simulink model "ResidualAware_TruckSim_Cosim"  (R2022b)
settings: Solver=FixedStepDiscrete  StartTime=0.0  StopTime=130  FixedStep=0.04  RelTol=1e-3
undefined symbols (not defined in the file or in its folder): ra_ego0, ra_P
settings Model: Creator=fjb  LastModifiedBy=fjb

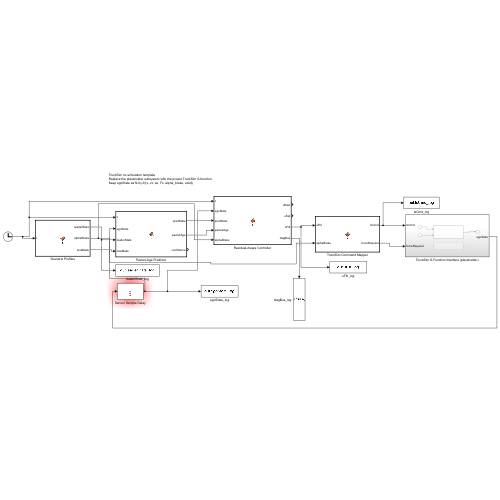
[thumbnail: Simulink's stored preview of the top-level diagram]
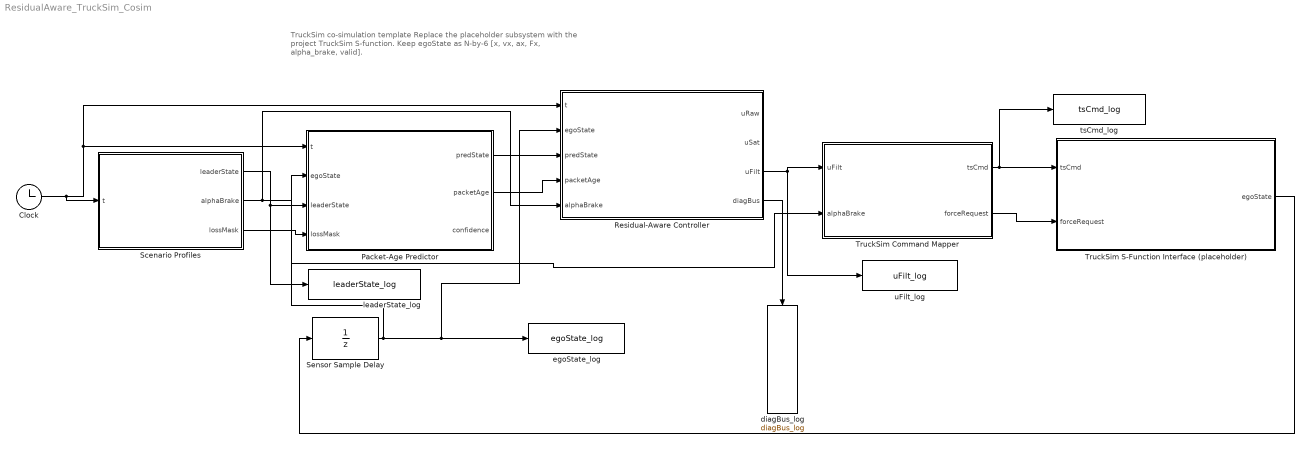
== system ResidualAware_TruckSim_Cosim ==
  note: TruckSim co-simulation template
      | Replace the placeholder subsystem with the project TruckSim S-function.
      | Keep egoState as N-by-6 [x, vx, ax, Fx, alpha_brake, valid].
  Clock : Clock
  Packet-Age Predictor : MATLAB Function  TreatAsAtomicUnit=on
  Residual-Aware Controller : MATLAB Function  TreatAsAtomicUnit=on
  Scenario Profiles : MATLAB Function  TreatAsAtomicUnit=on
  Sensor Sample Delay : UnitDelay  InitialCondition=ra_ego0  SampleTime=ra_P.Ts  HasFrameUpgradeWarning=on
  TruckSim Command Mapper : MATLAB Function  TreatAsAtomicUnit=on
  TruckSim S-Function Interface (placeholder) : Subsystem
  diagBus_log : ToWorkspace  VariableName=diagBus_log  SaveFormat=Structure With Time  SampleTime=-1
  egoState_log : ToWorkspace  VariableName=egoState_log  SaveFormat=Structure With Time  SampleTime=-1
  leaderState_log : ToWorkspace  VariableName=leaderState_log  SaveFormat=Structure With Time  SampleTime=-1
  tsCmd_log : ToWorkspace  VariableName=tsCmd_log  SaveFormat=Structure With Time  SampleTime=-1
  uFilt_log : ToWorkspace  VariableName=uFilt_log  SaveFormat=Structure With Time  SampleTime=-1
  wires:
  Clock/1 -> Packet-Age Predictor/1(t), Residual-Aware Controller/1(t), Scenario Profiles/1(t)
  Scenario Profiles/1(leaderState) -> Packet-Age Predictor/3(leaderState), leaderState_log/1
  Scenario Profiles/2(alphaBrake) -> Residual-Aware Controller/5(alphaBrake), TruckSim Command Mapper/2(alphaBrake)
  Scenario Profiles/3(lossMask) -> Packet-Age Predictor/4(lossMask)
  Sensor Sample Delay/1 -> Residual-Aware Controller/2(egoState), egoState_log/1, Packet-Age Predictor/2(egoState)
  Packet-Age Predictor/1(predState) -> Residual-Aware Controller/3(predState)
  Packet-Age Predictor/2(packetAge) -> Residual-Aware Controller/4(packetAge)
  Residual-Aware Controller/3(uFilt) -> uFilt_log/1, TruckSim Command Mapper/1(uFilt)
  Residual-Aware Controller/4(diagBus) -> diagBus_log/1
  TruckSim Command Mapper/1(tsCmd) -> TruckSim S-Function Interface (placeholder)/1(tsCmd), tsCmd_log/1
  TruckSim Command Mapper/2(forceRequest) -> TruckSim S-Function Interface (placeholder)/2(forceRequest)
  TruckSim S-Function Interface (placeholder)/1(egoState) -> Sensor Sample Delay/1

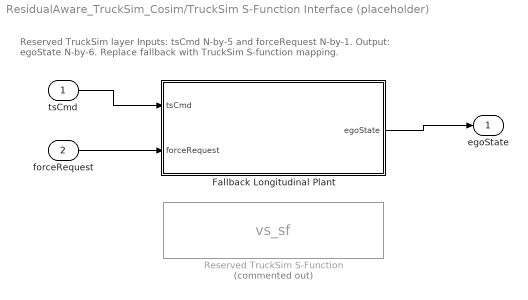
== system ResidualAware_TruckSim_Cosim/TruckSim S-Function Interface (placeholder) ==
  note: Reserved TruckSim layer
      | Inputs: tsCmd N-by-5 and forceRequest N-by-1.
      | Output: egoState N-by-6. Replace fallback with TruckSim S-function mapping.
  tsCmd : Inport
  forceRequest : Inport  Port=2
  Fallback Longitudinal Plant : MATLAB Function  TreatAsAtomicUnit=on
  Reserved TruckSim S-Function : S-Function  Commented=on  FunctionName=vs_sf  SFunctionDeploymentMode=off  EnableBusSupport=off
  egoState : Outport
  wires:
  tsCmd/1 -> Fallback Longitudinal Plant/1(tsCmd)
  forceRequest/1 -> Fallback Longitudinal Plant/2(forceRequest)
  Fallback Longitudinal Plant/1(egoState) -> egoState/1

== matlab function ResidualAware_TruckSim_Cosim/Packet-Age Predictor ==
  data: t input; predState output; egoState input; leaderState input; lossMask input; packetAge output; confidence output
function [predState, packetAge, confidence] = f(t, egoState, leaderState, lossMask)
%#codegen
coder.extrinsic('ra_params', 'ra_packet_predictor_step');
persistent lastPacket
predState = zeros(5, 5);
packetAge = zeros(5, 1);
confidence = zeros(5, 1);
if isempty(lastPacket)
    lastPacket = zeros(5, 5);
end
P = ra_params("compact5");
[predState, packetAge, confidence, lastPacket] = ra_packet_predictor_step(t, egoState, leaderState, lastPacket, lossMask, P);
end

== matlab function ResidualAware_TruckSim_Cosim/Scenario Profiles ==
  data: t input; leaderState output; alphaBrake output; lossMask output
function [leaderState, alphaBrake, lossMask] = f(t)
%#codegen
coder.extrinsic('ra_params', 'ra_leader_profile', 'ra_brake_fade_profile', 'ra_packet_loss_mask');
leaderState = zeros(1, 4);
alphaBrake = zeros(5, 1);
lossMask = false(5, 1);
P = ra_params("compact5");
leaderState = ra_leader_profile(t, P);
[alphaBrake, ~, ~] = ra_brake_fade_profile(t, P);
lossMask = ra_packet_loss_mask(t, P);
end

== matlab function ResidualAware_TruckSim_Cosim/Residual-Aware Controller ==
  data: t input; uRaw output; egoState input; predState input; packetAge input; alphaBrake input; uSat output; uFilt output; diagBus output
function [uRaw, uSat, uFilt, diagBus] = f(t, egoState, predState, packetAge, alphaBrake)
%#codegen
coder.extrinsic('ra_params', 'ra_init_controller_state', 'ra_controller_core');
persistent ctrlState
uRaw = zeros(5, 1);
uSat = zeros(5, 1);
uFilt = zeros(5, 1);
diagBus = zeros(5, 12);
P = ra_params("compact5");
if isempty(ctrlState)
    ctrlState = ra_init_controller_state(P);
end
[uRaw, uSat, uFilt, ctrlState, diagBus] = ra_controller_core(t, egoState, predState, packetAge, alphaBrake, ctrlState, P);
end

== matlab function ResidualAware_TruckSim_Cosim/TruckSim Command Mapper ==
  data: uFilt input; tsCmd output; alphaBrake input; forceRequest output
function [tsCmd, forceRequest] = f(uFilt, alphaBrake)
%#codegen
coder.extrinsic('ra_params', 'ra_trucksim_command_mapper');
tsCmd = zeros(5, 5);
forceRequest = zeros(5, 1);
P = ra_params("compact5");
[tsCmd, forceRequest] = ra_trucksim_command_mapper(uFilt, alphaBrake, P);
end

== matlab function ResidualAware_TruckSim_Cosim/TruckSim S-Function Interface (placeholder)/Fallback Longitudinal Plant ==
  data: tsCmd input; egoState output; forceRequest input
function egoState = f(tsCmd, forceRequest)
%#codegen
coder.extrinsic('ra_params', 'ra_fallback_trucksim_plant_step');
egoState = zeros(5, 6);
P = ra_params("compact5");
egoState = ra_fallback_trucksim_plant_step(tsCmd, forceRequest, P);
end
